simulink model "magball"  (R2020a)
settings: Solver=VariableStepAuto  StartTime=0.0  StopTime=10.0  RelTol=1e-3
settings Model: Creator=Shadman  LastModifiedBy=Shadman

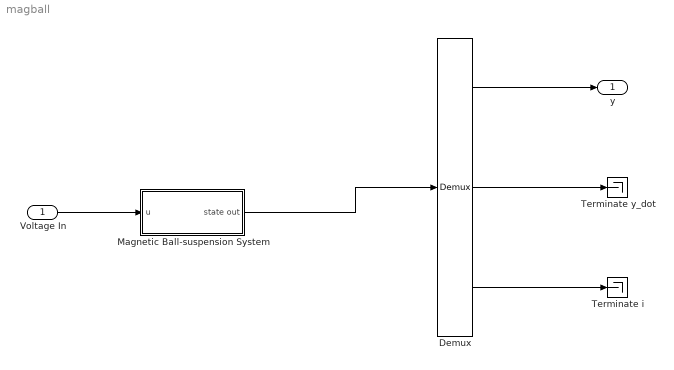
== system magball ==
  Voltage In : Inport
  Demux : Demux  Outputs=3
  Magnetic Ball-suspension System : Subsystem
  Terminate i : Terminator
  Terminate y_dot : Terminator
  y : Outport
  wires:
  Voltage In/1 -> Magnetic Ball-suspension System/1(u)
  Magnetic Ball-suspension System/1(state out) -> Demux/1
  Demux/1 -> y/1
  Demux/2 -> Terminate y_dot/1
  Demux/3 -> Terminate i/1

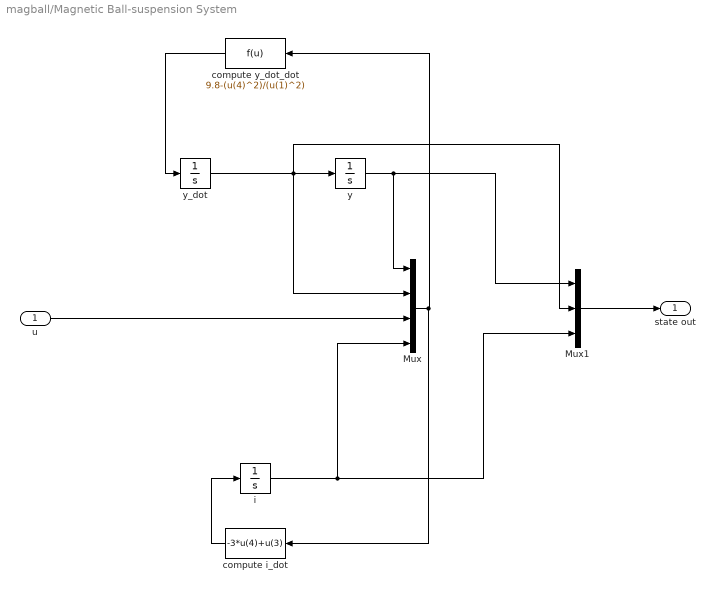
== system magball/Magnetic Ball-suspension System ==
  u : Inport
  Mux : Mux
  Mux1 : Mux  Inputs=3
  compute i_dot : Fcn  Expr=-3*u(4)+u(3)
  compute y_dot_dot : Fcn  Expr=9.8-(u(4)^2)/(u(1)^2)
  i : Integrator
  y : Integrator
  y_dot : Integrator
  state out : Outport  VectorParamsAs1DForOutWhenUnconnected=off
  wires:
  y/1 -> Mux/1, Mux1/1
  Mux/1 -> compute i_dot/1, compute y_dot_dot/1
  i/1 -> Mux/4, Mux1/3
  compute i_dot/1 -> i/1
  y_dot/1 -> Mux1/2, Mux/2, y/1
  compute y_dot_dot/1 -> y_dot/1
  Mux1/1 -> state out/1
  u/1 -> Mux/3
